simulink model "CM410B_SnsrMeasStrt"  (R2013b)
settings: Solver=FixedStepDiscrete  StartTime=0.0  StopTime=20  FixedStep=0.002  RelTol=1e-3
values from neighbouring files (symbols this model uses):
  ONEMICROSECCNT_CNT_U16 = DataDict.Constant    [CM410B_SnsrMeasStrt_DataDict.m]
  SnsrMeasStrtTrigDly = DataDict.Calibration    [CM410B_SnsrMeasStrt_DataDict.m]
libraries: simulink x2
settings Model: RequirementInfo={'doors' '00006115' '1' 'false' 'DOORS Surrogate Item' '' } %GIDa_184d7b6b_0c7e_41d3_b9a0_1a88eb3981d4  reqMgrSettings="100 S'doors','misc'{{S'surrogatepath','savemodel','savesurrogate','updateLinks','doorsLinks2sl','slLinks2Doors','purgeDoors','purgeSimulink','detaillevel','surrogateId','synctime'{{T\"/ESG Group/CM660A_HwTq1Meas\",M[1],M[1],M[0],M[0],M[1],M[0],M[0],M[1],T\"00006115\",T\"\"}},S'mode','pathStorage'{{T\"generic\",T\"modelRelative\"}}}}"  RecordCoverage=on  CovMetricSettings=dcmtrzoiw  CovFilter=CM700A_HwTq3Meas_covfilter  CovHTMLOptions=-sRT=1 -aTS=1 -bRG=1 -bTC=1 -hTR=0 -nFC=0 -scm=1 -bcm=1 -xEv=0  CovModelRefEnable=all  CovExternalEMLEnable=on  Creator=CZ68DS  LastModifiedBy=CZ68DS
settings SolverCC: AutoInsertRateTranBlk=on
settings DataIOCC: SaveFormat=StructureWithTime
settings OptimizationCC: BlockReduction=off  DefaultUnderspecifiedDataType=single  OptimizeBlockIOStorage=off  BufferReuse=off  ExpressionFolding=off  LocalBlockOutputs=off  OptimizeModelRefInitCode=on  LifeSpan=1
settings DebuggingCC: MultiTaskDSMMsg=warning  FrameProcessingCompatibilityMsg=error
settings HardwareCC: ProdIntDivRoundTo=Zero  ProdEndianess=LittleEndian  ProdHWDeviceType=Generic->Custom  TargetIntDivRoundTo=Zero  TargetEndianess=LittleEndian  TargetHWDeviceType=Generic->Custom
settings RTWCC: SystemTargetFile=ert.tlc  TemplateMakefile=ert_default_tmf  Description=Embedded Coder
settings CodeAppCC: IgnoreCustomStorageClasses=off
settings ERTTargetCC: CodeReplacementLibrary=C89/C90 (ANSI)  GenerateSampleERTMain=on  ERTCustomFileTemplate=example_file_process.tlc

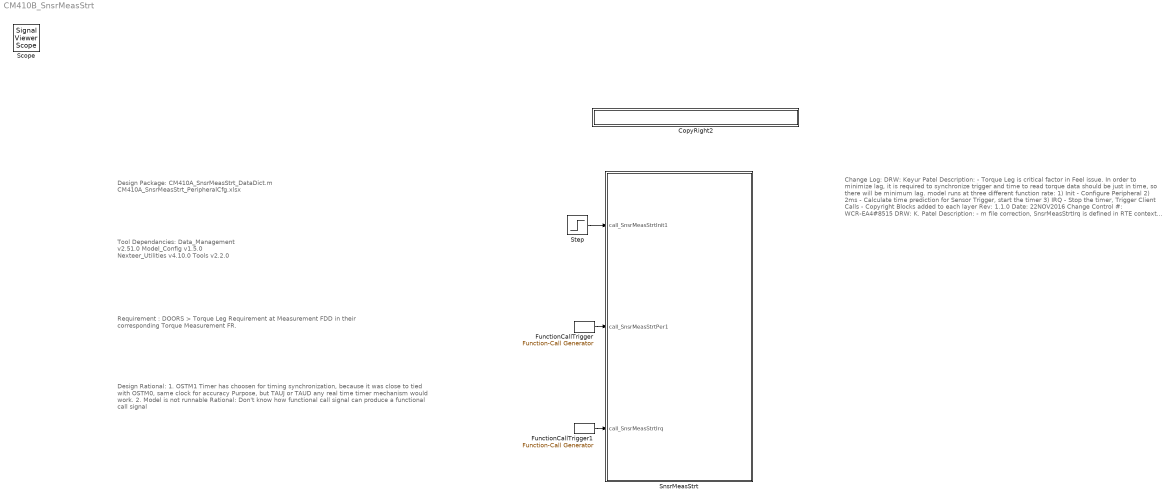
== system CM410B_SnsrMeasStrt ==
  note: Design Package:
      |
      | CM410A_SnsrMeasStrt_DataDict.m
      | CM410A_SnsrMeasStrt_PeripheralCfg.xlsx
  note: Change Log:
      |
      | DRW: Keyur Patel
      | Description:
      | - Torque Leg is critical factor in Feel issue. In order to minimize lag, it is required
      | to synchronize trigger and time to read torque data should be just in time, so there
      | will be minimum lag.
      |    model runs at three different function rate:
      |       1) Init - Configure Peripheral
      |       2) 2ms - Calculate time prediction for Sensor Trigger, start the timer
      |       3) IRQ - Stop the timer, Trigger Client Calls
      | - Copyright Blocks added to each layer
      |
      | Rev: 1.1.0
      | Date: 22NOV2016
      | Change Control #: WCR-EA4#8515
      | DRW: K. Patel
      | Description:
      | - m file correction, SnsrMeasStrtIrq is defined in RTE context and should be changed to Non-RTE.
      | - Remove OSTM register as Input / Output and define them as Ground / Terminate in Model.
      |
      | Rev: 1.0.0
      | Date: 23AUG2016
      | Change Control #: WCR-EA4#7052
      | DRW: K. Patel
      | Description:
      | - Baseline from CM410A Rev 1.1.0 - Initial Release
  note: Tool Dependancies:
      |
      | Data_Management v2.51.0
      | Model_Config v1.5.0
      | Nexteer_Utilities v4.10.0
      | Tools v2.2.0
  note: Requirement :
      |
      | DOORS >
      | Torque Leg Requirement at Measurement FDD in their
      | corresponding Torque Measurement FR.
  note: Design Rational:
      |
      | 1. OSTM1 Timer has choosen for timing synchronization,
      | because it was close to tied with OSTM0, same clock for accuracy
      | Purpose, but TAUJ or TAUD any real time timer mechanism would work.
      |
      | 2. Model is not runnable
      | Rational: Don't know how functional call signal can produce a functional call signal
  CopyRight2 : Subsystem  Description=|  mask(Copyright Information){none=on}
      | Copyright info block.                                               
      |                                                                     
      | Place copyright information at the top of every subsystem in design.
      mask prompts: none "No parameters"
      mask help: Place copyright information at the top of every subsystem in design.
      mask Display:
      | NxtrConf = 'Nexteer Confidential';
      | 
      | sys = bdroot; %handle for the current model ("system")
      | first = get_param(sys,'Created');
      | first = first(end-3:end);  %year is last four digits
      | 
      | last = get_param(sys,'LastModifiedDate');
      | if isempty(last)
      |     last = datestr(now,'yyyy');
      | else
      |     last = last(end-3:end);
      | end
      | 
      | if strcmp(first,last)
      |     fprintf('%s -- Copyright %s Nexteer',NxtrConf,first)
      | else
      |     fprintf('%s -- %s%s- %s Nexteer',NxtrConf,char(169),first,last)
      | end
  FunctionCallTrigger : simulink/Ports & Subsystems/Function-Call Generator  RequirementInfo={} %GIDa_461051ca_e299_4da2_91c0_e73e41056377  sample_time=0.002  numberOfIterations=1
      settings: AttributesFormatString=%<sample_time>
  FunctionCallTrigger1 : simulink/Ports & Subsystems/Function-Call Generator  RequirementInfo={} %GIDa_438cb3ad_bac1_4c45_9e8e_a890b08ea603  sample_time=0.002  numberOfIterations=1
      settings: AttributesFormatString=%<sample_time>
  SnsrMeasStrt : Subsystem  RequirementInfo={} %GIDa_76d712c1_5f1a_450e_83af_7c4f481758f4
  Step : Step  Before=1  After=0  SampleTime=0
  Scope : SignalViewerScope  IOType=viewer  SampleTime=-1  ZoomMode=on
      settings: TimeRange=auto  TickLabels=OneTimeTick  LimitDataPoints=on  SaveToWorkspace=off  SaveName=ScopeData  YMin=-10  YMax=10  SampleInput=off
  wires:
  FunctionCallTrigger/1 -> SnsrMeasStrt/2(call_SnsrMeasStrtPer1)
  Step/1 -> SnsrMeasStrt/1(call_SnsrMeasStrtInit1)
  FunctionCallTrigger1/1 -> SnsrMeasStrt/3(call_SnsrMeasStrtIrq)

== system CM410B_SnsrMeasStrt/CopyRight2 ==

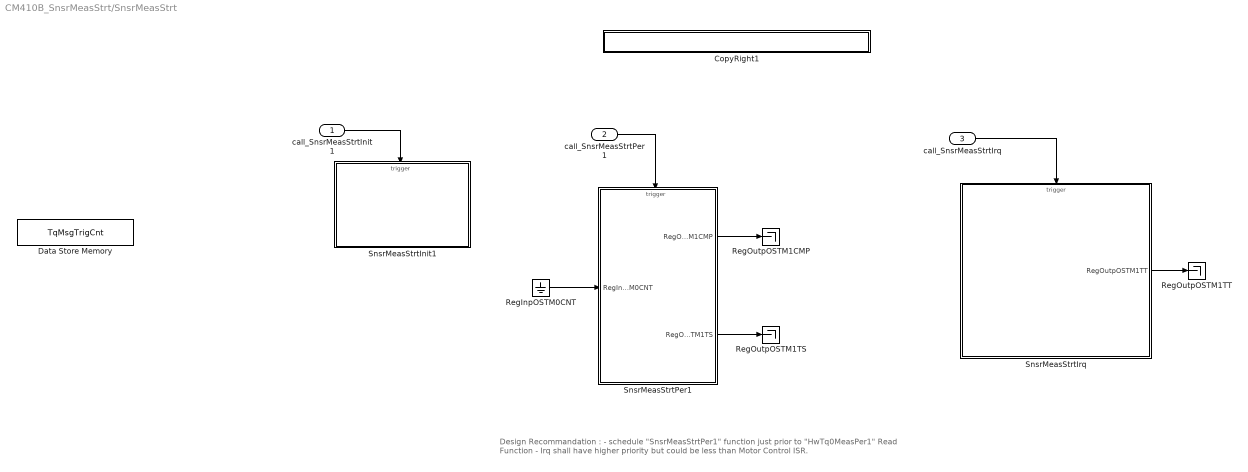
== system CM410B_SnsrMeasStrt/SnsrMeasStrt ==
  note: Design Recommandation :
      |
      | - schedule "SnsrMeasStrtPer1" function just prior to "HwTq0MeasPer1" Read Function
      | - Irq shall have higher priority but could be less than Motor Control ISR.
  call_SnsrMeasStrtInit1 : Inport
  call_SnsrMeasStrtPer1 : Inport  Description=2ms  Port=2
      settings: AttributesFormatString=%<Description>
  call_SnsrMeasStrtIrq : Inport  Description=IRQ  Port=3
      settings: AttributesFormatString=%<Description>
  CopyRight1 : Subsystem  Description=|  mask(Copyright Information){none=on}
      | Copyright info block.                                               
      |                                                                     
      | Place copyright information at the top of every subsystem in design.
      mask prompts: none "No parameters"
      mask help: Place copyright information at the top of every subsystem in design.
      mask Display:
      | NxtrConf = 'Nexteer Confidential';
      | 
      | sys = bdroot; %handle for the current model ("system")
      | first = get_param(sys,'Created');
      | first = first(end-3:end);  %year is last four digits
      | 
      | last = get_param(sys,'LastModifiedDate');
      | if isempty(last)
      |     last = datestr(now,'yyyy');
      | else
      |     last = last(end-3:end);
      | end
      | 
      | if strcmp(first,last)
      |     fprintf('%s -- Copyright %s Nexteer',NxtrConf,first)
      | else
      |     fprintf('%s -- %s%s- %s Nexteer',NxtrConf,char(169),first,last)
      | end
  Data Store Memory : DataStoreMemory  DataStoreName=TqMsgTrigCnt  ReadBeforeWriteMsg=warning  WriteAfterWriteMsg=warning  WriteAfterReadMsg=warning  ShowAdditionalParam=off  StateMustResolveToSignalObject=on
  RegInpOSTM0CNT : Ground
  RegOutpOSTM1CMP : Terminator
  RegOutpOSTM1TS : Terminator
  RegOutpOSTM1TT : Terminator
  SnsrMeasStrtInit1 : Subsystem  TreatAsAtomicUnit=on
  SnsrMeasStrtIrq : Subsystem  RequirementInfo={} %GIDa_ac2e4248_233e_47e7_8dc6_e55969fb5c4e  TreatAsAtomicUnit=on
  SnsrMeasStrtPer1 : Subsystem  RequirementInfo={} %GIDa_31b3da74_5937_4fb2_b915_5c5c5e5711e7  TreatAsAtomicUnit=on
  wires:
  call_SnsrMeasStrtPer1/1 -> SnsrMeasStrtPer1/Trigger
  call_SnsrMeasStrtInit1/1 -> SnsrMeasStrtInit1/Trigger
  SnsrMeasStrtPer1/1(RegOutpOSTM1CMP) -> RegOutpOSTM1CMP/1
  SnsrMeasStrtPer1/2(RegOutpOSTM1TS) -> RegOutpOSTM1TS/1
  call_SnsrMeasStrtIrq/1 -> SnsrMeasStrtIrq/Trigger
  RegInpOSTM0CNT/1 -> SnsrMeasStrtPer1/1(RegInpOSTM0CNT)
  SnsrMeasStrtIrq/1(RegOutpOSTM1TT) -> RegOutpOSTM1TT/1

== system CM410B_SnsrMeasStrt/SnsrMeasStrt/CopyRight1 ==

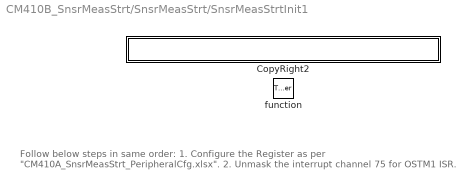
== system CM410B_SnsrMeasStrt/SnsrMeasStrt/SnsrMeasStrtInit1 ==
  note: Follow below steps in same order:
      |
      | 1. Configure the Register as per  "CM410A_SnsrMeasStrt_PeripheralCfg.xlsx".
      | 2. Unmask the interrupt channel 75 for OSTM1 ISR.
  function : TriggerPort  TriggerType=falling
  CopyRight2 : Subsystem  Description=|  mask(Copyright Information){none=on}
      | Copyright info block.                                               
      |                                                                     
      | Place copyright information at the top of every subsystem in design.
      mask prompts: none "No parameters"
      mask help: Place copyright information at the top of every subsystem in design.
      mask Display:
      | NxtrConf = 'Nexteer Confidential';
      | 
      | sys = bdroot; %handle for the current model ("system")
      | first = get_param(sys,'Created');
      | first = first(end-3:end);  %year is last four digits
      | 
      | last = get_param(sys,'LastModifiedDate');
      | if isempty(last)
      |     last = datestr(now,'yyyy');
      | else
      |     last = last(end-3:end);
      | end
      | 
      | if strcmp(first,last)
      |     fprintf('%s -- Copyright %s Nexteer',NxtrConf,first)
      | else
      |     fprintf('%s -- %s%s- %s Nexteer',NxtrConf,char(169),first,last)
      | end

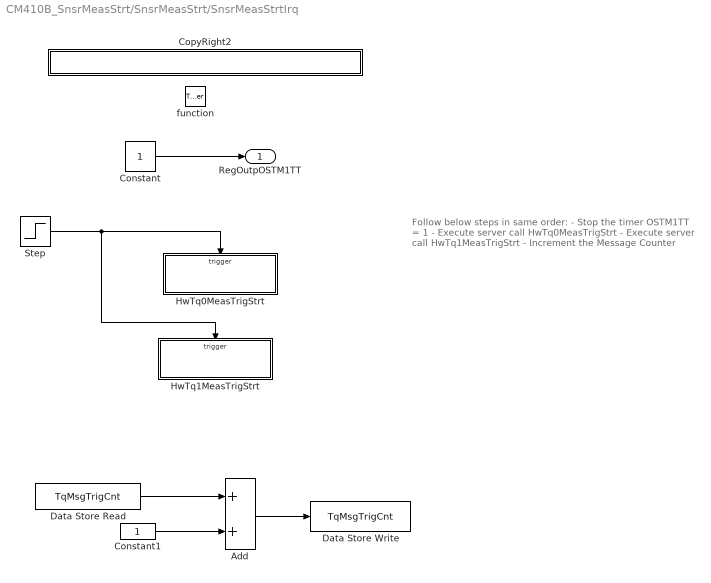
== system CM410B_SnsrMeasStrt/SnsrMeasStrt/SnsrMeasStrtIrq ==
  note: Follow below steps in same order:
      |
      | - Stop the timer OSTM1TT = 1
      | - Execute server call HwTq0MeasTrigStrt
      | - Execute server call HwTq1MeasTrigStrt
      | - Increment the Message Counter
  function : TriggerPort  TriggerType=function-call
  Add : Sum
  Constant : Constant
  Constant1 : Constant
  CopyRight2 : Subsystem  Description=|  mask(Copyright Information){none=on}
      | Copyright info block.                                               
      |                                                                     
      | Place copyright information at the top of every subsystem in design.
      mask prompts: none "No parameters"
      mask help: Place copyright information at the top of every subsystem in design.
      mask Display:
      | NxtrConf = 'Nexteer Confidential';
      | 
      | sys = bdroot; %handle for the current model ("system")
      | first = get_param(sys,'Created');
      | first = first(end-3:end);  %year is last four digits
      | 
      | last = get_param(sys,'LastModifiedDate');
      | if isempty(last)
      |     last = datestr(now,'yyyy');
      | else
      |     last = last(end-3:end);
      | end
      | 
      | if strcmp(first,last)
      |     fprintf('%s -- Copyright %s Nexteer',NxtrConf,first)
      | else
      |     fprintf('%s -- %s%s- %s Nexteer',NxtrConf,char(169),first,last)
      | end
  Data Store Read : DataStoreRead  DataStoreName=TqMsgTrigCnt
  Data Store Write : DataStoreWrite  DataStoreName=TqMsgTrigCnt
  HwTq0MeasTrigStrt : Subsystem  RequirementInfo={} %GIDa_9f56f688_e0dd_47c4_b71c_91650712956b  TreatAsAtomicUnit=on
  HwTq1MeasTrigStrt : Subsystem  RequirementInfo={} %GIDa_a4940c02_cf7a_4948_a0ea_eca2fa84041c  Priority=10  TreatAsAtomicUnit=on
  Step : Step  Before=1  After=0  SampleTime=0
  RegOutpOSTM1TT : Outport
  wires:
  Step/1 -> HwTq1MeasTrigStrt/Trigger, HwTq0MeasTrigStrt/Trigger
  Constant/1 -> RegOutpOSTM1TT/1
  Constant1/1 -> Add/2
  Add/1 -> Data Store Write/1
  Data Store Read/1 -> Add/1

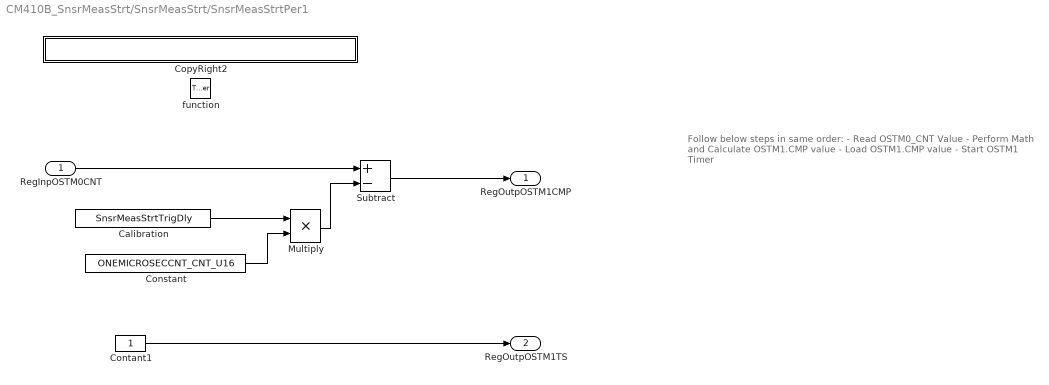
== system CM410B_SnsrMeasStrt/SnsrMeasStrt/SnsrMeasStrtPer1 ==
  note: Follow below steps in same order:
      |
      | - Read OSTM0_CNT Value
      | - Perform Math and Calculate OSTM1.CMP value
      | - Load OSTM1.CMP value
      | - Start OSTM1 Timer
  RegInpOSTM0CNT : Inport
  function : TriggerPort  TriggerType=function-call
  "Calibration " : Constant  Value=SnsrMeasStrtTrigDly  VectorParams1D=off
  Constant : Constant  Value=ONEMICROSECCNT_CNT_U16
  Contant1 : Constant
  CopyRight2 : Subsystem  Description=|  mask(Copyright Information){none=on}
      | Copyright info block.                                               
      |                                                                     
      | Place copyright information at the top of every subsystem in design.
      mask prompts: none "No parameters"
      mask help: Place copyright information at the top of every subsystem in design.
      mask Display:
      | NxtrConf = 'Nexteer Confidential';
      | 
      | sys = bdroot; %handle for the current model ("system")
      | first = get_param(sys,'Created');
      | first = first(end-3:end);  %year is last four digits
      | 
      | last = get_param(sys,'LastModifiedDate');
      | if isempty(last)
      |     last = datestr(now,'yyyy');
      | else
      |     last = last(end-3:end);
      | end
      | 
      | if strcmp(first,last)
      |     fprintf('%s -- Copyright %s Nexteer',NxtrConf,first)
      | else
      |     fprintf('%s -- %s%s- %s Nexteer',NxtrConf,char(169),first,last)
      | end
  Multiply : Product  Inputs=**
  Subtract : Sum  Inputs=+-
  RegOutpOSTM1CMP : Outport  RequirementInfo={} %GIDa_3b2abd0f_dff5_44f3_b788_adb2172836f5
  RegOutpOSTM1TS : Outport  RequirementInfo={} %GIDa_5eff5979_1038_44df_a727_ac7fcfb158b0  Port=2
  wires:
  RegInpOSTM0CNT/1 -> Subtract/1
  "Calibration "/1 -> Multiply/1
  Constant/1 -> Multiply/2
  Multiply/1 -> Subtract/2
  Subtract/1 -> RegOutpOSTM1CMP/1
  Contant1/1 -> RegOutpOSTM1TS/1

== system CM410B_SnsrMeasStrt/SnsrMeasStrt/SnsrMeasStrtInit1/CopyRight2 ==

== system CM410B_SnsrMeasStrt/SnsrMeasStrt/SnsrMeasStrtIrq/CopyRight2 ==

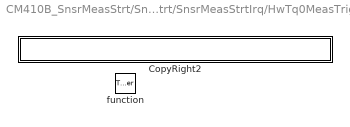
== system CM410B_SnsrMeasStrt/SnsrMeasStrt/SnsrMeasStrtIrq/HwTq0MeasTrigStrt ==
  function : TriggerPort  TriggerType=falling
  CopyRight2 : Subsystem  Description=|  mask(Copyright Information){none=on}
      | Copyright info block.                                               
      |                                                                     
      | Place copyright information at the top of every subsystem in design.
      mask prompts: none "No parameters"
      mask help: Place copyright information at the top of every subsystem in design.
      mask Display:
      | NxtrConf = 'Nexteer Confidential';
      | 
      | sys = bdroot; %handle for the current model ("system")
      | first = get_param(sys,'Created');
      | first = first(end-3:end);  %year is last four digits
      | 
      | last = get_param(sys,'LastModifiedDate');
      | if isempty(last)
      |     last = datestr(now,'yyyy');
      | else
      |     last = last(end-3:end);
      | end
      | 
      | if strcmp(first,last)
      |     fprintf('%s -- Copyright %s Nexteer',NxtrConf,first)
      | else
      |     fprintf('%s -- %s%s- %s Nexteer',NxtrConf,char(169),first,last)
      | end

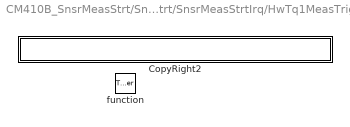
== system CM410B_SnsrMeasStrt/SnsrMeasStrt/SnsrMeasStrtIrq/HwTq1MeasTrigStrt ==
  function : TriggerPort  TriggerType=falling
  CopyRight2 : Subsystem  Description=|  mask(Copyright Information){none=on}
      | Copyright info block.                                               
      |                                                                     
      | Place copyright information at the top of every subsystem in design.
      mask prompts: none "No parameters"
      mask help: Place copyright information at the top of every subsystem in design.
      mask Display:
      | NxtrConf = 'Nexteer Confidential';
      | 
      | sys = bdroot; %handle for the current model ("system")
      | first = get_param(sys,'Created');
      | first = first(end-3:end);  %year is last four digits
      | 
      | last = get_param(sys,'LastModifiedDate');
      | if isempty(last)
      |     last = datestr(now,'yyyy');
      | else
      |     last = last(end-3:end);
      | end
      | 
      | if strcmp(first,last)
      |     fprintf('%s -- Copyright %s Nexteer',NxtrConf,first)
      | else
      |     fprintf('%s -- %s%s- %s Nexteer',NxtrConf,char(169),first,last)
      | end

== system CM410B_SnsrMeasStrt/SnsrMeasStrt/SnsrMeasStrtPer1/CopyRight2 ==

== system CM410B_SnsrMeasStrt/SnsrMeasStrt/SnsrMeasStrtIrq/HwTq0MeasTrigStrt/CopyRight2 ==

== system CM410B_SnsrMeasStrt/SnsrMeasStrt/SnsrMeasStrtIrq/HwTq1MeasTrigStrt/CopyRight2 ==
